simulink library "Tank_bib"  (R2017b)
settings: Solver=ode45  StartTime=0.0  StopTime=10.0  RelTol=1e-3  EnableMultiTasking=on
undefined symbols (not defined in the file or in its folder): National_Instruments, PCI
libraries: simulink x22, sldrtlib x3, vrlib x2
settings Model: Creator=andreasj  LastModifiedBy=Oliver
settings DataIOCC: LimitDataPoints=on  SaveFormat=Array
settings OptimizationCC: LifeSpan=inf
settings DebuggingCC: SFUnexpectedBacktrackingDiag=warning  SFNoUnconditionalDefaultTransitionDiag=warning  SFExecutionAtInitializationDiag=none
settings HardwareCC: ProdBitPerPointer=32  ProdBitPerSizeT=32  ProdBitPerPtrDiffT=32  ProdLargestAtomicFloat=None  ProdIntDivRoundTo=Undefined  ProdEndianess=Unspecified  ProdWordSize=32  ProdHWDeviceType=32-bit Generic
settings ModelReferenceCC: PropagateSignalLabelsOutOfModel=off
settings CodeAppCC: StateflowObjectComments=on
settings GRTTargetCC: TargetLangStandard=C89/C90 (ANSI)  GeneratePreprocessorConditionals=Disable all
settings ConfigComp: CovMetricSettings=dw  CovHtmlReporting=on  CovSaveCumulativeToWorkspaceVar=on  CovSaveSingleToWorkspaceVar=on  CovExternalEMLEnable=off

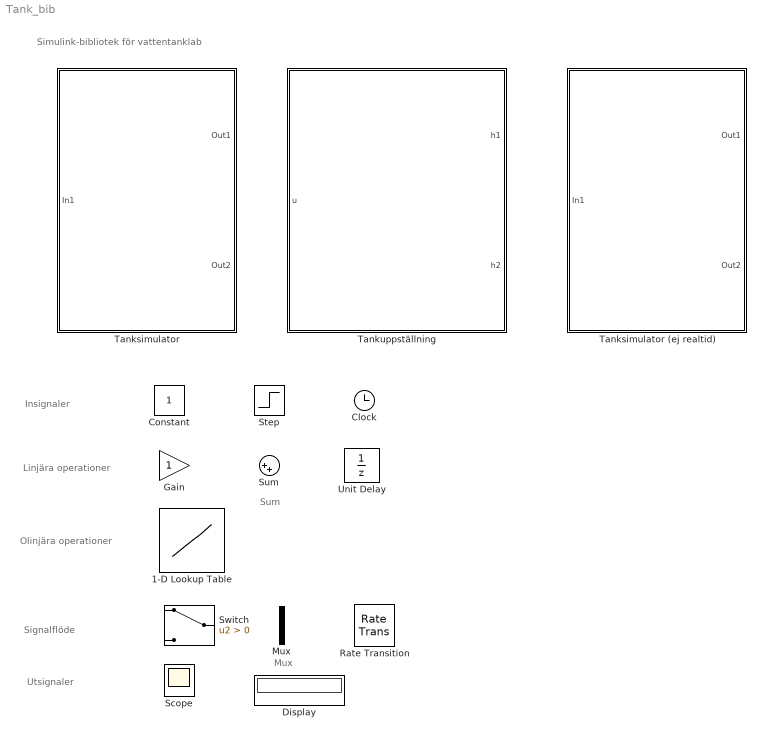
== system Tank_bib ==
  note: Mux
  note: Sum
  note: Utsignaler
  note: Signalflöde
  note: Olinjära operationer
  note: Linjära operationer
  note: Insignaler
  note: Simulink-bibliotek för vattentanklab
  1-D Lookup Table : Lookup_n-D  NumberOfTableDimensions=1  BreakpointsForDimension1=[-5:5]  Table=tanh([-5:5])  InternalRulePriority=Speed  RndMeth=Simplest  InputSameDT=on
  Clock : Clock
  Constant : Constant
  Display : Display
  Gain : Gain
  Mux : Mux  Inputs=2
  Rate Transition : RateTransition
  Scope : Scope
  Step : Step  SampleTime=0
  Sum : Sum  Inputs=|++
  Switch : Switch  Criteria=u2 > Threshold
  Tanksimulator : Subsystem  mask{valve_opening=0.0, plug=off}
      mask prompts: valve_opening "Handventil öppen grader"; plug "Utlopp pluggat"
      mask init:
      | R=3.4;
      | k=22;
      | alpha=.35;
      | a1=0.171;
      | a2=0.169;
      | A=pi*R^2;
      | H=3.2;
      | g=982;
      mask Display: image(imread('Tanks.png'))
  Tanksimulator (ej realtid) : Subsystem  AncestorBlock=Tank_bib/Tanksimulator  mask{valve_opening=0.0, plug=off}
      mask prompts: valve_opening "Handventil öppen grader"; plug "Utlopp pluggat"
      mask init:
      | R=3.4;
      | k=22;
      | alpha=.35;
      | a1=0.171;
      | a2=0.169;
      | A=pi*R^2;
      | H=3.2;
      | g=982;
      mask Display: image(imread('Tanks.png'))
  Tankuppställning : Subsystem  StopFcn=|  mask(Realtime interface for the tank process){ts=0.02}
      | dtsys = find_system(bdroot(gcs),'masktype','Realtime interface for the tank process');
      | chn = get_param([dtsys{1},'/Analog Output'],'Channels');                              
      | s = daq.createSession('ni');                                                          
      | channel = ['ao',chn-1];                                                               
      | s.addAnalogOutputChannel('Dev1', channel, 'Voltage');                                 
      | x = zeros(5,1);                                                                       
      | s.queueOutputData(x);                                                                 
      | lh = s.addlistener('DataRequired', ...                                                
      | @(src,event) src.queueOutputData(x));                                                 
      | s.startBackground();                                                                  
      | s.wait();                                                                             
      | s.stop();                                                                             
      | delete(lh);                                                                           
      | clear chn;                                                                            
      | clear s;                                                                              
      | clear channel;                                                                        
      | clear lh;                                                                             
      | clear x;
      mask prompts: ts "Sample time"
      mask help:
      | This block represents the physical interface from the computer to the tank process.
      |
      | The input u is the voltage that is provided for the pump, the output h1 is the measured level in the upper tank in [V] and the output h2 is the
      | measured level in the lower tank in [V].
      |
      | You need to provide the sample rate at which the voltage to the pump is updated and the level measurements are sampled. The sample rate should not be less than 0.02 seconds.
      mask Display: image(imread('tank_icon.jpg'))
  Unit Delay : UnitDelay  SampleTime=-1

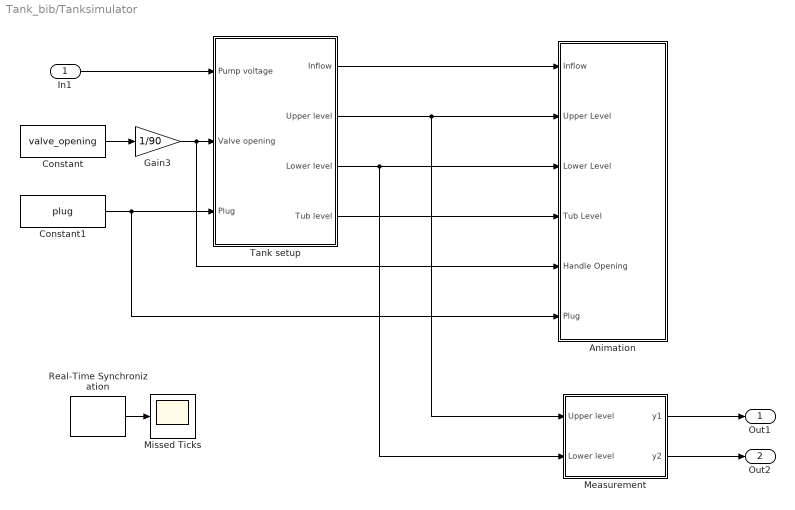
== system Tank_bib/Tanksimulator ==
  In1 : Inport
  Animation : Subsystem
  Constant : Constant  Value=valve_opening
  Constant1 : Constant  Value=plug
  Gain3 : Gain  Gain=1/90
  Measurement : Subsystem
  Missed Ticks : Scope
  Real-Time Synchronization : sldrtlib/Real-Time Synchronization  SampleTime=0.05  MaxMissedTicks=1000  ShowMissedTicks=on  YieldWhenWaiting=off
  Tank setup : Subsystem
  Out1 : Outport
  Out2 : Outport  Port=2
  wires:
  Real-Time Synchronization/1 -> Missed Ticks/1
  Gain3/1 -> Tank setup/2(Valve opening), Animation/5(Handle Opening)
  Constant/1 -> Gain3/1
  Constant1/1 -> Tank setup/3(Plug), Animation/6(Plug)
  Tank setup/1(Inflow) -> Animation/1(Inflow)
  Tank setup/2(Upper level) -> Measurement/1(Upper level), Animation/2(Upper Level)
  Tank setup/3(Lower level) -> Measurement/2(Lower level), Animation/3(Lower Level)
  Tank setup/4(Tub level) -> Animation/4(Tub Level)
  Measurement/1(y1) -> Out1/1
  Measurement/2(y2) -> Out2/1
  In1/1 -> Tank setup/1(Pump voltage)

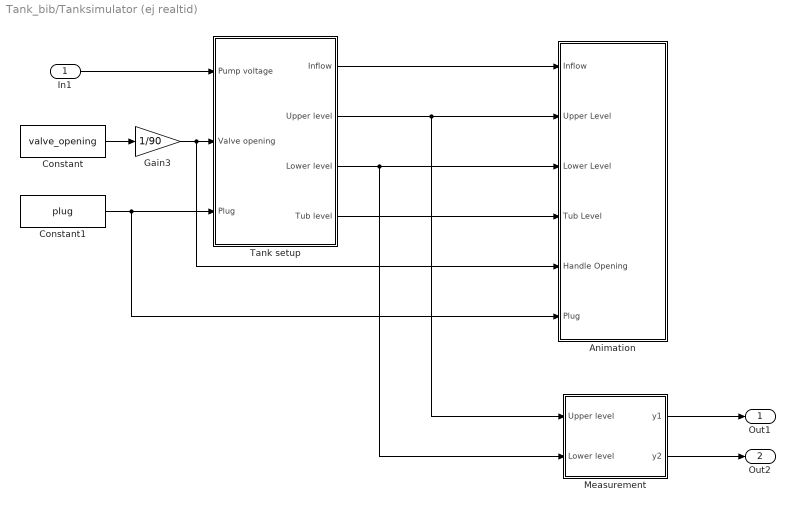
== system Tank_bib/Tanksimulator (ej realtid) ==
  In1 : Inport
  Animation : Subsystem
  Constant : Constant  Value=valve_opening
  Constant1 : Constant  Value=plug
  Gain3 : Gain  Gain=1/90
  Measurement : Subsystem
  Tank setup : Subsystem
  Out1 : Outport
  Out2 : Outport  Port=2
  wires:
  Gain3/1 -> Tank setup/2(Valve opening), Animation/5(Handle Opening)
  Constant/1 -> Gain3/1
  Constant1/1 -> Tank setup/3(Plug), Animation/6(Plug)
  Tank setup/1(Inflow) -> Animation/1(Inflow)
  Tank setup/2(Upper level) -> Measurement/1(Upper level), Animation/2(Upper Level)
  Tank setup/3(Lower level) -> Measurement/2(Lower level), Animation/3(Lower Level)
  Tank setup/4(Tub level) -> Animation/4(Tub Level)
  Measurement/1(y1) -> Out1/1
  Measurement/2(y2) -> Out2/1
  In1/1 -> Tank setup/1(Pump voltage)

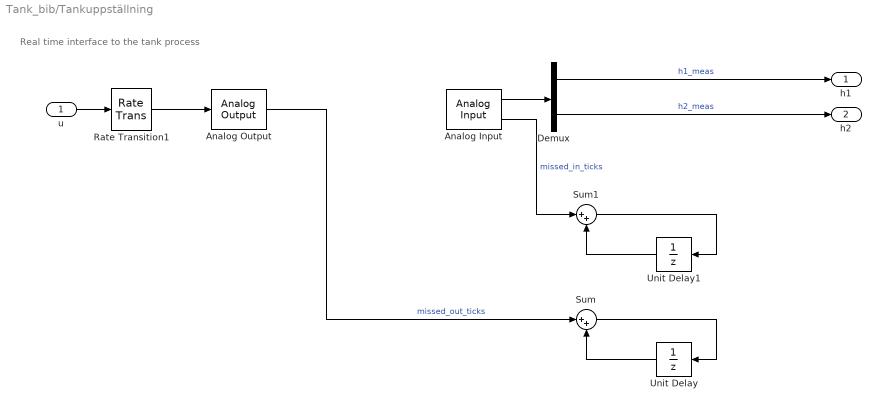
== system Tank_bib/Tankuppställning ==
  note: Real time interface to the tank process
  u : Inport
  Analog Input : sldrtlib/Analog Input  SampleTime=ts  MaxMissedTicks=500000000  ShowMissedTicks=on  YieldWhenWaiting=off  DrvName=National_Instruments/PCI-6024E  DrvAddress=4294967295  DrvOptions=[0 0 0 0 0 0]  Channels=1:2  RangeMode=1  VoltRange=1  DataType=1
      settings: AttributesFormatString=National Instruments\nPCI-6024E [auto]  SourceProductName=Simulink Desktop Real-Time
  Analog Output : sldrtlib/Analog Output  SampleTime=ts  MaxMissedTicks=500000000  ShowMissedTicks=on  YieldWhenWaiting=off  DrvName=National_Instruments/PCI-6024E  DrvAddress=4294967295  DrvOptions=[0 0 0 0 0 0]  Channels=1  RangeMode=1  VoltRange=1  InitialValue=0  FinalValue=0
      settings: AttributesFormatString=National Instruments\nPCI-6024E [auto]  SourceProductName=Simulink Desktop Real-Time
  Demux : Demux  Outputs=2
  Rate Transition1 : RateTransition  OutPortSampleTime=ts
  Sum : Sum  Inputs=|++
  Sum1 : Sum  Inputs=|++
  Unit Delay : UnitDelay  SampleTime=-1
  Unit Delay1 : UnitDelay  SampleTime=-1
  h1 : Outport
  h2 : Outport  Port=2
  wires:
  Sum1/1 -> Unit Delay1/1
  Unit Delay1/1 -> Sum1/2
  Sum/1 -> Unit Delay/1
  Unit Delay/1 -> Sum/2
  Analog Input/2 -> Sum1/1  "missed_in_ticks"
  Demux/2 -> h2/1  "h2_meas"
  Demux/1 -> h1/1  "h1_meas"
  Analog Input/1 -> Demux/1
  Analog Output/1 -> Sum/1  "missed_out_ticks"
  u/1 -> Rate Transition1/1
  Rate Transition1/1 -> Analog Output/1

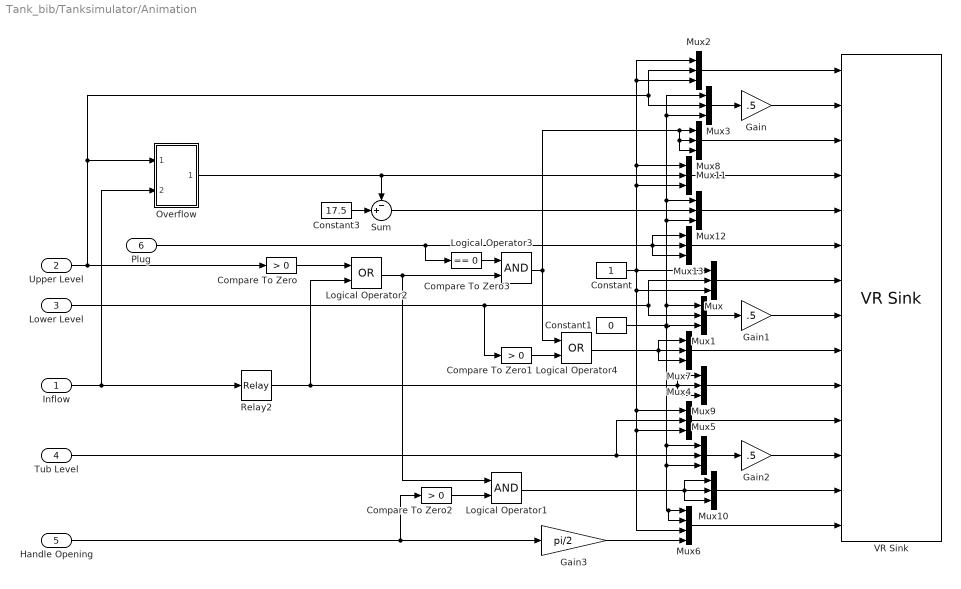
== system Tank_bib/Tanksimulator/Animation ==
  Inflow : Inport
  Upper Level : Inport  Port=2
  Lower Level : Inport  Port=3
  Tub Level : Inport  Port=4
  Handle Opening : Inport  Port=5
  Plug : Inport  Port=6
  Compare To Zero : simulink/Logic and Bit Operations/Compare To Zero  relop=>  OutDataTypeStr=boolean
  Compare To Zero1 : simulink/Logic and Bit Operations/Compare To Zero  relop=>  OutDataTypeStr=boolean
  Compare To Zero2 : simulink/Logic and Bit Operations/Compare To Zero  relop=>  OutDataTypeStr=boolean
  Compare To Zero3 : simulink/Logic and Bit Operations/Compare To Zero  relop===  OutDataTypeStr=boolean
  Constant : Constant
  Constant1 : Constant  Value=0
  Constant3 : Constant  Value=17.5
  Gain : Gain  Gain=.5
  Gain1 : Gain  Gain=.5
  Gain2 : Gain  Gain=.5
  Gain3 : Gain  Gain=pi/2
  Logical Operator1 : Logic  AllPortsSameDT=off  OutDataTypeStr=boolean
  Logical Operator2 : Logic  Operator=OR  AllPortsSameDT=off  OutDataTypeStr=boolean
  Logical Operator3 : Logic  AllPortsSameDT=off  OutDataTypeStr=boolean
  Logical Operator4 : Logic  Operator=OR  AllPortsSameDT=off  OutDataTypeStr=boolean
  Mux{,1..5,7..13} (13 alike) : Mux  Inputs=3
  Mux6 : Mux
  Overflow : Subsystem
  Relay2 : Relay
  Sum : Sum  Inputs=-+|
  VR Sink : vrlib/VR Sink  InstantiateOnLoad=on  SampleTime=0.1  ViewEnable=on  RemoteChange=off  RemoteView=off  FieldsWritten=Water1.scale.3.1.1.double#Water1.translation.3.1.1.double#Flow1.scale.3.1.1.double#OverFlow1.scale.3.1.1.double#OverFlow1.translation.3.1.1.double#Plug.scale.3.1.1.double#Water2.scale.3.1.1.double#Water2.translation.3.1.1.double#Flow2.scale.3.1.1.double#Inflow.scale.3.1.1.double#TubWater.scale.3.1.1.double#TubWater.translation.3.1.1.double#DisturbanceFlow.scale.3.1.1.double#Handle.rotation.4.1.1.double  WorldFileName=Tank_world.wrl  AutoView=on  VideoDimensions=[]  AllowVariableSize=off
      settings: SourceProductBaseCode=VR
  wires:
  Overflow/1(Out1) -> Mux11/2, Sum/1
  Mux13/1 -> VR Sink/6
  Mux6/1 -> VR Sink/14
  Mux10/1 -> VR Sink/13
  Gain2/1 -> VR Sink/12
  Mux4/1 -> VR Sink/11
  Mux9/1 -> VR Sink/10
  Mux7/1 -> VR Sink/9
  Gain1/1 -> VR Sink/8
  Mux/1 -> VR Sink/7
  Mux12/1 -> VR Sink/5
  Mux11/1 -> VR Sink/4
  Mux8/1 -> VR Sink/3
  Gain/1 -> VR Sink/2
  Mux2/1 -> VR Sink/1
  Compare To Zero1/1 -> Logical Operator4/2
  Compare To Zero3/1 -> Logical Operator3/1
  Logical Operator3/1 -> Logical Operator4/1, Mux8/1, Mux8/2, Mux8/3
  Plug/1 -> Compare To Zero3/1, Mux13/2, Mux13/1, Mux13/3
  Upper Level/1 -> Compare To Zero/1, Mux3/2, Mux2/2, Overflow/1(In1)
  Mux1/1 -> Gain1/1
  Mux5/1 -> Gain2/1
  Tub Level/1 -> Mux4/2, Mux5/2
  Inflow/1 -> Relay2/1, Overflow/2(In2)
  Constant/1 -> Mux6/3, Mux4/3, Mux4/1, Mux/3, Mux2/1, Mux2/3, Mux11/1, Mux11/3, Mux/1
  Lower Level/1 -> Compare To Zero1/1, Mux/2, Mux1/2
  Constant1/1 -> Mux6/2, Mux6/1, Mux5/3, Mux5/1, Mux1/3, Mux3/1, Mux3/3, Mux12/1, Mux12/3, Mux1/1
  Mux3/1 -> Gain/1
  Logical Operator4/1 -> Mux7/3, Mux7/2, Mux7/1
  Relay2/1 -> Mux9/3, Mux9/1, Mux9/2, Logical Operator2/2
  Logical Operator1/1 -> Mux10/2, Mux10/1, Mux10/3
  Handle Opening/1 -> Gain3/1, Compare To Zero2/1
  Gain3/1 -> Mux6/4
  Sum/1 -> Mux12/2
  Constant3/1 -> Sum/2
  Compare To Zero/1 -> Logical Operator2/1
  Compare To Zero2/1 -> Logical Operator1/2
  Logical Operator2/1 -> Logical Operator3/2, Logical Operator1/1

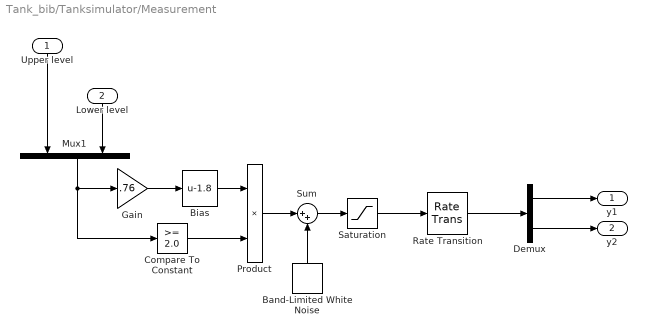
== system Tank_bib/Tanksimulator/Measurement ==
  Upper level : Inport
  Lower level : Inport  Port=2
  Band-Limited White Noise : simulink/Sources/Band-Limited White Noise  Cov=[0.00001 0.00001]  Ts=0.1  seed=[23341 23342]
  Bias : Bias  Bias=-1.8
  Compare To Constant : simulink/Logic and Bit Operations/Compare To Constant  relop=>=  const=2.0  OutDataTypeStr=boolean
  Demux : Demux  Outputs=2
  Gain : Gain  Gain=.76
  Mux1 : Mux  Inputs=2
  Product : Product
  Rate Transition : RateTransition  OutPortSampleTime=0.02
  Saturation : Saturate  UpperLimit=10  LowerLimit=0
  Sum : Sum  Inputs=|++
  y1 : Outport
  y2 : Outport  Port=2
  wires:
  Gain/1 -> Bias/1
  Mux1/1 -> Gain/1, Compare To Constant/1
  Bias/1 -> Product/1
  Sum/1 -> Saturation/1
  Product/1 -> Sum/1
  Band-Limited White Noise/1 -> Sum/2
  Saturation/1 -> Rate Transition/1
  Compare To Constant/1 -> Product/2
  Demux/1 -> y1/1
  Lower level/1 -> Mux1/2
  Demux/2 -> y2/1
  Upper level/1 -> Mux1/1
  Rate Transition/1 -> Demux/1

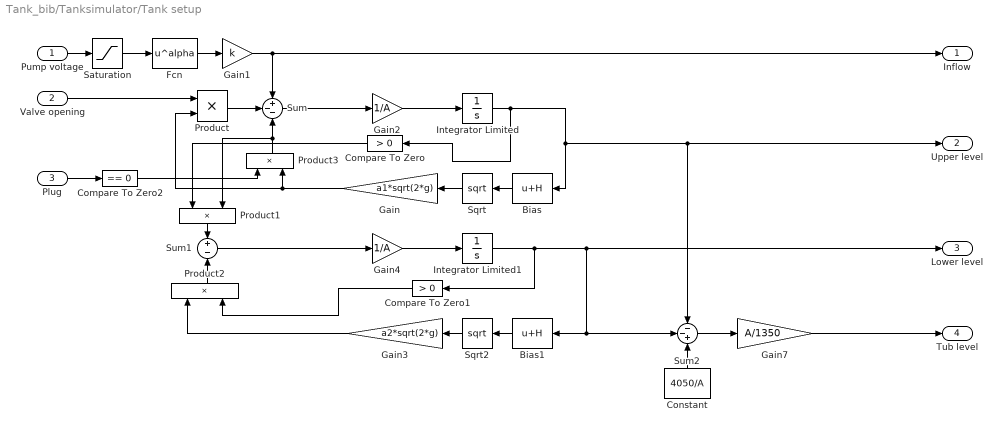
== system Tank_bib/Tanksimulator/Tank setup ==
  Pump voltage : Inport
  Valve opening : Inport  Port=2
  Plug : Inport  Port=3
  Bias : Bias  Bias=H
  Bias1 : Bias  Bias=H
  Compare To Zero : simulink/Logic and Bit Operations/Compare To Zero  relop=>  OutDataTypeStr=boolean
  Compare To Zero1 : simulink/Logic and Bit Operations/Compare To Zero  relop=>  OutDataTypeStr=boolean
  Compare To Zero2 : simulink/Logic and Bit Operations/Compare To Zero  relop===  OutDataTypeStr=boolean
  Constant : Constant  Value=4050/A
  Fcn : Fcn  Expr=u^alpha
  Gain : Gain  Gain=a1*sqrt(2*g)
  Gain1 : Gain  Gain=k
  Gain2 : Gain  Gain=1/A
  Gain3 : Gain  Gain=a2*sqrt(2*g)
  Gain4 : Gain  Gain=1/A
  Gain7 : Gain  Gain=A/1350
  Integrator Limited : Integrator  LimitOutput=on  UpperSaturationLimit=17.5  LowerSaturationLimit=0
  Integrator Limited1 : Integrator  LimitOutput=on  UpperSaturationLimit=17.5  LowerSaturationLimit=0
  Product{,1..3} (4 alike) : Product
  Saturation : Saturate  UpperLimit=10  LowerLimit=0
  Sqrt : Sqrt  SaturateOnIntegerOverflow=on
  Sqrt2 : Sqrt  SaturateOnIntegerOverflow=on
  Sum : Sum  Inputs=+--
  Sum1 : Sum  Inputs=+|-
  Sum2 : Sum  Inputs=--+
  Inflow : Outport
  Upper level : Outport  Port=2
  Lower level : Outport  Port=3
  Tub level : Outport  Port=4
  wires:
  Product3/1 -> Product1/2, Sum/3
  Compare To Zero2/1 -> Product3/1
  Plug/1 -> Compare To Zero2/1
  Gain3/1 -> Product2/1
  Gain/1 -> Product/2, Product3/2
  Integrator Limited1/1 -> Compare To Zero1/1, Lower level/1, Sum2/2, Bias1/1
  Constant/1 -> Sum2/3
  Fcn/1 -> Gain1/1
  Gain4/1 -> Integrator Limited1/1
  Compare To Zero1/1 -> Product2/2
  Product2/1 -> Sum1/2
  Gain1/1 -> Sum/1, Inflow/1
  Gain7/1 -> Tub level/1
  Bias/1 -> Sqrt/1
  Integrator Limited/1 -> Compare To Zero/1, Upper level/1, Sum2/1, Bias/1
  Sum2/1 -> Gain7/1
  Sqrt2/1 -> Gain3/1
  Sum1/1 -> Gain4/1
  Bias1/1 -> Sqrt2/1
  Sum/1 -> Gain2/1
  Pump voltage/1 -> Saturation/1
  Product/1 -> Sum/2
  Gain2/1 -> Integrator Limited/1
  Sqrt/1 -> Gain/1
  Valve opening/1 -> Product/1
  Compare To Zero/1 -> Product1/1
  Product1/1 -> Sum1/1
  Saturation/1 -> Fcn/1

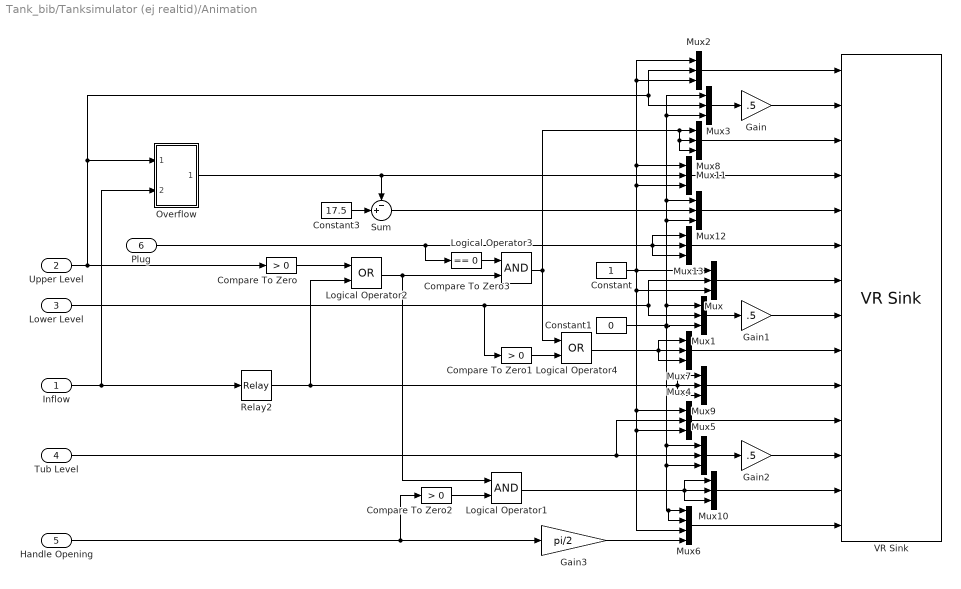
== system Tank_bib/Tanksimulator (ej realtid)/Animation ==
  Inflow : Inport
  Upper Level : Inport  Port=2
  Lower Level : Inport  Port=3
  Tub Level : Inport  Port=4
  Handle Opening : Inport  Port=5
  Plug : Inport  Port=6
  Compare To Zero : simulink/Logic and Bit Operations/Compare To Zero  relop=>  OutDataTypeStr=boolean
  Compare To Zero1 : simulink/Logic and Bit Operations/Compare To Zero  relop=>  OutDataTypeStr=boolean
  Compare To Zero2 : simulink/Logic and Bit Operations/Compare To Zero  relop=>  OutDataTypeStr=boolean
  Compare To Zero3 : simulink/Logic and Bit Operations/Compare To Zero  relop===  OutDataTypeStr=boolean
  Constant : Constant
  Constant1 : Constant  Value=0
  Constant3 : Constant  Value=17.5
  Gain : Gain  Gain=.5
  Gain1 : Gain  Gain=.5
  Gain2 : Gain  Gain=.5
  Gain3 : Gain  Gain=pi/2
  Logical Operator1 : Logic  AllPortsSameDT=off  OutDataTypeStr=boolean
  Logical Operator2 : Logic  Operator=OR  AllPortsSameDT=off  OutDataTypeStr=boolean
  Logical Operator3 : Logic  AllPortsSameDT=off  OutDataTypeStr=boolean
  Logical Operator4 : Logic  Operator=OR  AllPortsSameDT=off  OutDataTypeStr=boolean
  Mux{,1..5,7..13} (13 alike) : Mux  Inputs=3
  Mux6 : Mux
  Overflow : Subsystem
  Relay2 : Relay
  Sum : Sum  Inputs=-+|
  VR Sink : vrlib/VR Sink  InstantiateOnLoad=on  SampleTime=0.1  ViewEnable=on  RemoteChange=off  RemoteView=off  FieldsWritten=Water1.scale.3.1.1.double#Water1.translation.3.1.1.double#Flow1.scale.3.1.1.double#OverFlow1.scale.3.1.1.double#OverFlow1.translation.3.1.1.double#Plug.scale.3.1.1.double#Water2.scale.3.1.1.double#Water2.translation.3.1.1.double#Flow2.scale.3.1.1.double#Inflow.scale.3.1.1.double#TubWater.scale.3.1.1.double#TubWater.translation.3.1.1.double#DisturbanceFlow.scale.3.1.1.double#Handle.rotation.4.1.1.double  WorldFileName=Tank_world.wrl  AutoView=on  VideoDimensions=[]  AllowVariableSize=off
      settings: SourceProductBaseCode=VR
  wires:
  Overflow/1(Out1) -> Mux11/2, Sum/1
  Mux13/1 -> VR Sink/6
  Mux6/1 -> VR Sink/14
  Mux10/1 -> VR Sink/13
  Gain2/1 -> VR Sink/12
  Mux4/1 -> VR Sink/11
  Mux9/1 -> VR Sink/10
  Mux7/1 -> VR Sink/9
  Gain1/1 -> VR Sink/8
  Mux/1 -> VR Sink/7
  Mux12/1 -> VR Sink/5
  Mux11/1 -> VR Sink/4
  Mux8/1 -> VR Sink/3
  Gain/1 -> VR Sink/2
  Mux2/1 -> VR Sink/1
  Compare To Zero1/1 -> Logical Operator4/2
  Compare To Zero3/1 -> Logical Operator3/1
  Logical Operator3/1 -> Logical Operator4/1, Mux8/1, Mux8/2, Mux8/3
  Plug/1 -> Compare To Zero3/1, Mux13/2, Mux13/1, Mux13/3
  Upper Level/1 -> Compare To Zero/1, Mux3/2, Mux2/2, Overflow/1(In1)
  Mux1/1 -> Gain1/1
  Mux5/1 -> Gain2/1
  Tub Level/1 -> Mux4/2, Mux5/2
  Inflow/1 -> Relay2/1, Overflow/2(In2)
  Constant/1 -> Mux6/3, Mux4/3, Mux4/1, Mux/3, Mux2/1, Mux2/3, Mux11/1, Mux11/3, Mux/1
  Lower Level/1 -> Compare To Zero1/1, Mux/2, Mux1/2
  Constant1/1 -> Mux6/2, Mux6/1, Mux5/3, Mux5/1, Mux1/3, Mux3/1, Mux3/3, Mux12/1, Mux12/3, Mux1/1
  Mux3/1 -> Gain/1
  Logical Operator4/1 -> Mux7/3, Mux7/2, Mux7/1
  Relay2/1 -> Mux9/3, Mux9/1, Mux9/2, Logical Operator2/2
  Logical Operator1/1 -> Mux10/2, Mux10/1, Mux10/3
  Handle Opening/1 -> Gain3/1, Compare To Zero2/1
  Gain3/1 -> Mux6/4
  Sum/1 -> Mux12/2
  Constant3/1 -> Sum/2
  Compare To Zero/1 -> Logical Operator2/1
  Compare To Zero2/1 -> Logical Operator1/2
  Logical Operator2/1 -> Logical Operator3/2, Logical Operator1/1

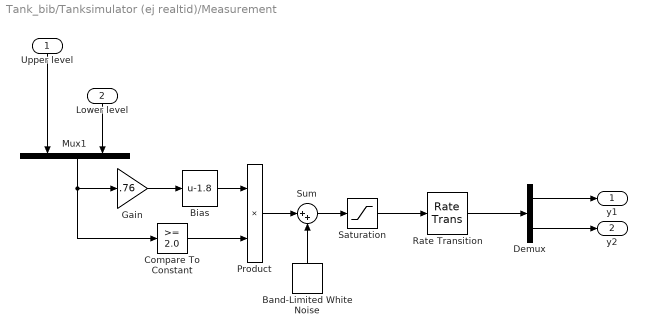
== system Tank_bib/Tanksimulator (ej realtid)/Measurement ==
  Upper level : Inport
  Lower level : Inport  Port=2
  Band-Limited White Noise : simulink/Sources/Band-Limited White Noise  Cov=[0.00001 0.00001]  Ts=0.1  seed=[23341 23342]
  Bias : Bias  Bias=-1.8
  Compare To Constant : simulink/Logic and Bit Operations/Compare To Constant  relop=>=  const=2.0  OutDataTypeStr=boolean
  Demux : Demux  Outputs=2
  Gain : Gain  Gain=.76
  Mux1 : Mux  Inputs=2
  Product : Product
  Rate Transition : RateTransition  OutPortSampleTime=0.02
  Saturation : Saturate  UpperLimit=10  LowerLimit=0
  Sum : Sum  Inputs=|++
  y1 : Outport
  y2 : Outport  Port=2
  wires:
  Gain/1 -> Bias/1
  Mux1/1 -> Gain/1, Compare To Constant/1
  Bias/1 -> Product/1
  Sum/1 -> Saturation/1
  Product/1 -> Sum/1
  Band-Limited White Noise/1 -> Sum/2
  Saturation/1 -> Rate Transition/1
  Compare To Constant/1 -> Product/2
  Demux/1 -> y1/1
  Lower level/1 -> Mux1/2
  Demux/2 -> y2/1
  Upper level/1 -> Mux1/1
  Rate Transition/1 -> Demux/1

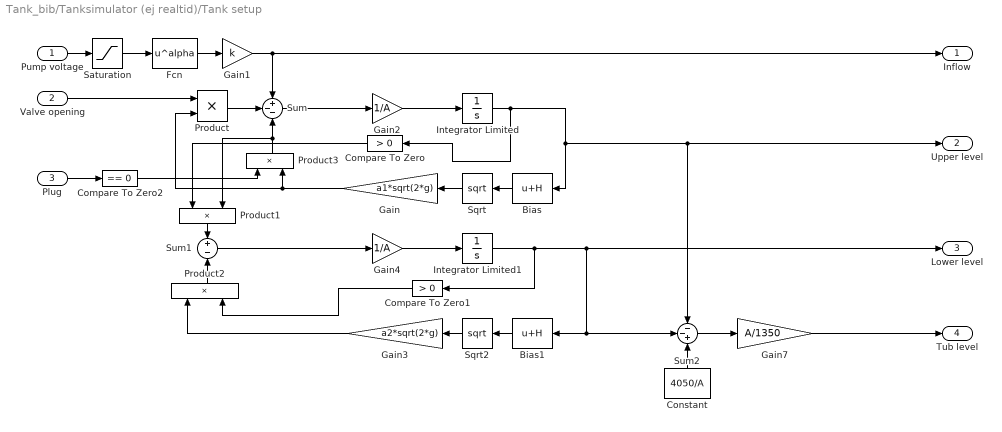
== system Tank_bib/Tanksimulator (ej realtid)/Tank setup ==
  Pump voltage : Inport
  Valve opening : Inport  Port=2
  Plug : Inport  Port=3
  Bias : Bias  Bias=H
  Bias1 : Bias  Bias=H
  Compare To Zero : simulink/Logic and Bit Operations/Compare To Zero  relop=>  OutDataTypeStr=boolean
  Compare To Zero1 : simulink/Logic and Bit Operations/Compare To Zero  relop=>  OutDataTypeStr=boolean
  Compare To Zero2 : simulink/Logic and Bit Operations/Compare To Zero  relop===  OutDataTypeStr=boolean
  Constant : Constant  Value=4050/A
  Fcn : Fcn  Expr=u^alpha
  Gain : Gain  Gain=a1*sqrt(2*g)
  Gain1 : Gain  Gain=k
  Gain2 : Gain  Gain=1/A
  Gain3 : Gain  Gain=a2*sqrt(2*g)
  Gain4 : Gain  Gain=1/A
  Gain7 : Gain  Gain=A/1350
  Integrator Limited : Integrator  LimitOutput=on  UpperSaturationLimit=17.5  LowerSaturationLimit=0
  Integrator Limited1 : Integrator  LimitOutput=on  UpperSaturationLimit=17.5  LowerSaturationLimit=0
  Product{,1..3} (4 alike) : Product
  Saturation : Saturate  UpperLimit=10  LowerLimit=0
  Sqrt : Sqrt  SaturateOnIntegerOverflow=on
  Sqrt2 : Sqrt  SaturateOnIntegerOverflow=on
  Sum : Sum  Inputs=+--
  Sum1 : Sum  Inputs=+|-
  Sum2 : Sum  Inputs=--+
  Inflow : Outport
  Upper level : Outport  Port=2
  Lower level : Outport  Port=3
  Tub level : Outport  Port=4
  wires:
  Product3/1 -> Product1/2, Sum/3
  Compare To Zero2/1 -> Product3/1
  Plug/1 -> Compare To Zero2/1
  Gain3/1 -> Product2/1
  Gain/1 -> Product/2, Product3/2
  Integrator Limited1/1 -> Compare To Zero1/1, Lower level/1, Sum2/2, Bias1/1
  Constant/1 -> Sum2/3
  Fcn/1 -> Gain1/1
  Gain4/1 -> Integrator Limited1/1
  Compare To Zero1/1 -> Product2/2
  Product2/1 -> Sum1/2
  Gain1/1 -> Sum/1, Inflow/1
  Gain7/1 -> Tub level/1
  Bias/1 -> Sqrt/1
  Integrator Limited/1 -> Compare To Zero/1, Upper level/1, Sum2/1, Bias/1
  Sum2/1 -> Gain7/1
  Sqrt2/1 -> Gain3/1
  Sum1/1 -> Gain4/1
  Bias1/1 -> Sqrt2/1
  Sum/1 -> Gain2/1
  Pump voltage/1 -> Saturation/1
  Product/1 -> Sum/2
  Gain2/1 -> Integrator Limited/1
  Sqrt/1 -> Gain/1
  Valve opening/1 -> Product/1
  Compare To Zero/1 -> Product1/1
  Product1/1 -> Sum1/1
  Saturation/1 -> Fcn/1

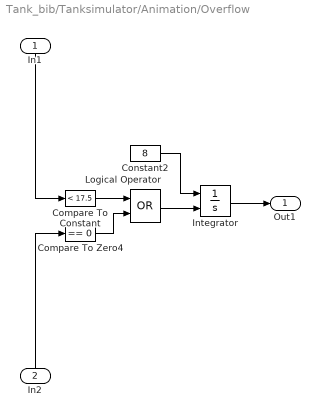
== system Tank_bib/Tanksimulator/Animation/Overflow ==
  In1 : Inport
  In2 : Inport  Port=2
  Compare To Constant : simulink/Logic and Bit Operations/Compare To Constant  relop=<  const=17.5  OutDataTypeStr=boolean
  Compare To Zero4 : simulink/Logic and Bit Operations/Compare To Zero  relop===  OutDataTypeStr=boolean
  Constant2 : Constant  Value=8
  Integrator : Integrator  ExternalReset=level hold  WrapState=on  WrappedStateUpperValue=9  WrappedStateLowerValue=0
  Logical Operator : Logic  Operator=OR  AllPortsSameDT=off  OutDataTypeStr=boolean
  Out1 : Outport
  wires:
  Integrator/1 -> Out1/1
  Logical Operator/1 -> Integrator/2
  Constant2/1 -> Integrator/1
  In1/1 -> Compare To Constant/1
  In2/1 -> Compare To Zero4/1
  Compare To Constant/1 -> Logical Operator/1
  Compare To Zero4/1 -> Logical Operator/2

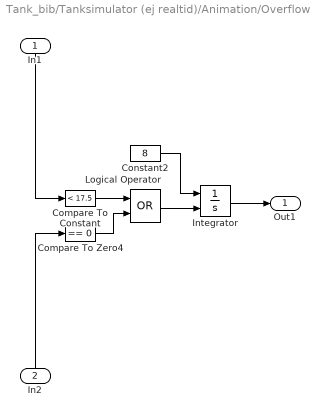
== system Tank_bib/Tanksimulator (ej realtid)/Animation/Overflow ==
  In1 : Inport
  In2 : Inport  Port=2
  Compare To Constant : simulink/Logic and Bit Operations/Compare To Constant  relop=<  const=17.5  OutDataTypeStr=boolean
  Compare To Zero4 : simulink/Logic and Bit Operations/Compare To Zero  relop===  OutDataTypeStr=boolean
  Constant2 : Constant  Value=8
  Integrator : Integrator  ExternalReset=level hold  WrapState=on  WrappedStateUpperValue=9  WrappedStateLowerValue=0
  Logical Operator : Logic  Operator=OR  AllPortsSameDT=off  OutDataTypeStr=boolean
  Out1 : Outport
  wires:
  Integrator/1 -> Out1/1
  Logical Operator/1 -> Integrator/2
  Constant2/1 -> Integrator/1
  In1/1 -> Compare To Constant/1
  In2/1 -> Compare To Zero4/1
  Compare To Constant/1 -> Logical Operator/1
  Compare To Zero4/1 -> Logical Operator/2
